simulink model "Arm_Simulation"  (R2022b)
settings: Solver=ode23t  StartTime=0.0  StopTime=10  RelTol=1e-3
undefined symbols (not defined in the file or in its folder): alpha, LF, Ts, X, Y, Z
libraries: sm_lib x16, nesl_utility x8, spsEdgeDetectorLib x6, instrumentseriallib x3, simulink_extras x3, simulink x2, svdutilitieslib x1
(part 2 of 2)

== matlab function Arm_Simulation/Path Planning/Non-Adaptive Primitive/Vertical Polynomial ==
  data: p output; t input; r_o parameter; T_swing input; beta parameter
function p = fcn(t, r_o, T_swing, beta)

T_arch = T_swing / 2;

if t <= T_arch
    % Swing Phase - Liftoff: Quintic Polynomial 1
    c0 = 0;
    c1 = 0;
    c2 = 0;
    c3 = 10 / T_arch^3;
    c4 = -15 / T_arch^4;
    c5 = 6 / T_arch^5;
    
    C = [c0; c1; c2; c3; c4; c5];
    T = [1, t, t^2, t^3, t^4, t^5];

    p = r_o*T*C;
elseif t <= T_swing
    % Swing Phase - Touchdown: Quintic Polynomial 2
    c0 = 1;
    c1 = 0;
    c2 = 0;
    c3 = -10 / T_arch^3;
    c4 = 15 / T_arch^4;
    c5 = -6 / T_arch^5;
    
    C = [c0; c1; c2; c3; c4; c5];

    t = t - T_arch;

    T = [1, t, t^2, t^3, t^4, t^5];

    p = r_o*T*C;
else
    % Stance Phase: Zero
    p = 0;
end

== matlab function Arm_Simulation/Path Planning/Non-Adaptive Primitive/Horizontal Polynomial ==
  data: p output; t input; r_o parameter; T_swing input; beta parameter
function p = fcn(t, r_o, T_swing, beta)

v = -2*r_o / beta;

offset = 2*r_o - v*T_swing;

c0 = -r_o;
c1 = v;
c2 = 0;
c3 = 10 * offset / T_swing^3;
c4 = -15 * offset / T_swing^4;
c5 = 6 * offset / T_swing^5;

C = [c0; c1; c2; c3; c4; c5];
T = [1, t, t^2, t^3, t^4, t^5];

p = T*C;

== matlab function Arm_Simulation/Path Planning/Adaptive Primitive/Vertical/Liftoff Polynomial ==
  data: p output; t input; r_o parameter; T_up input; z input
function p = fcn(t, r_o, T_up, z)

p = (r_o - z);

c0 = z;
c1 = 0;
c2 = 0;
c3 = p * 10 / T_up^3;
c4 = -p * 15 / T_up^4;
c5 = p * 6 / T_up^5;

C = [c0; c1; c2; c3; c4; c5];
T = [1, t, t^2, t^3, t^4, t^5];

p = T*C;

== matlab function Arm_Simulation/Path Planning/Adaptive Primitive/Vertical/Touchdown Polynomial ==
  data: T_up output; p output; t input; r_o parameter; delta input; beta parameter
function [T_up, p] = fcn(t, r_o, delta, beta)

T_down = (1 - beta) / 2;
T_up = T_down + delta;

% Swing Phase - Touchdown: Quintic Polynomial 2
c0 = 1;
c1 = 0;
c2 = 0;
c3 = -10 / T_down^3;
c4 = 15 / T_down^4;
c5 = -6 / T_down^5;

C = [c0; c1; c2; c3; c4; c5];

t = t - T_up;

T = [1, t, t^2, t^3, t^4, t^5];

p = r_o*T*C;

== matlab function Arm_Simulation/FK Sim/DH Row 2 ==
  data: theta input; d input; alpha input; T output; a input
function T = fcn(theta, d, alpha, a)

ct = cos(theta);
st = sin(theta);
ca = cos(alpha);
sa = sin(alpha);

T = [    ct,   -st,    0,      a;
      st*ca,  ct*ca, -sa,  -sa*d;
      st*sa,  ct*sa,  ca,   ca*d;
          0,      0,    0,      1];
end

== matlab function Arm_Simulation/FK Sim/DH Row 1 ==
  data: theta input; d input; alpha input; T output; a input
function T = fcn(theta, d, alpha, a)

ct = cos(theta);
st = sin(theta);
ca = cos(alpha);
sa = sin(alpha);

T = [    ct,   -st,    0,      a;
      st*ca,  ct*ca, -sa,  -sa*d;
      st*sa,  ct*sa,  ca,   ca*d;
          0,      0,    0,      1];
end

== matlab function Arm_Simulation/FK Sim/DH Row 3 ==
  data: theta input; d input; alpha input; T output; a input
function T = fcn(theta, d, alpha, a)

ct = cos(theta);
st = sin(theta);
ca = cos(alpha);
sa = sin(alpha);

T = [    ct,   -st,    0,      a;
      st*ca,  ct*ca, -sa,  -sa*d;
      st*sa,  ct*sa,  ca,   ca*d;
          0,      0,    0,      1];
end

== matlab function Arm_Simulation/FK Sim/DH Row 4 ==
  data: theta input; d input; alpha input; T output; a input
function T = fcn(theta, d, alpha, a)

ct = cos(theta);
st = sin(theta);
ca = cos(alpha);
sa = sin(alpha);

T = [    ct,   -st,    0,      a;
      st*ca,  ct*ca, -sa,  -sa*d;
      st*sa,  ct*sa,  ca,   ca*d;
          0,      0,    0,      1];
end

== matlab function Arm_Simulation/FK Sim1/DH Row 1 ==
  data: theta input; d input; alpha input; T output; a input
function T = fcn(theta, d, alpha, a)

ct = cos(theta);
st = sin(theta);
ca = cos(alpha);
sa = sin(alpha);

T = [    ct,   -st,    0,      a;
      st*ca,  ct*ca, -sa,  -sa*d;
      st*sa,  ct*sa,  ca,   ca*d;
          0,      0,    0,      1];
end

== matlab function Arm_Simulation/FK Sim1/DH Row 2 ==
  data: theta input; d input; alpha input; T output; a input
function T = fcn(theta, d, alpha, a)

ct = cos(theta);
st = sin(theta);
ca = cos(alpha);
sa = sin(alpha);

T = [    ct,   -st,    0,      a;
      st*ca,  ct*ca, -sa,  -sa*d;
      st*sa,  ct*sa,  ca,   ca*d;
          0,      0,    0,      1];
end

== matlab function Arm_Simulation/FK Sim1/DH Row 3 ==
  data: theta input; d input; alpha input; T output; a input
function T = fcn(theta, d, alpha, a)

ct = cos(theta);
st = sin(theta);
ca = cos(alpha);
sa = sin(alpha);

T = [    ct,   -st,    0,      a;
      st*ca,  ct*ca, -sa,  -sa*d;
      st*sa,  ct*sa,  ca,   ca*d;
          0,      0,    0,      1];
end

== matlab function Arm_Simulation/FK Sim1/DH Row 4 ==
  data: theta input; d input; alpha input; T output; a input
function T = fcn(theta, d, alpha, a)

ct = cos(theta);
st = sin(theta);
ca = cos(alpha);
sa = sin(alpha);

T = [    ct,   -st,    0,      a;
      st*ca,  ct*ca, -sa,  -sa*d;
      st*sa,  ct*sa,  ca,   ca*d;
          0,      0,    0,      1];
end

== matlab function Arm_Simulation/Path Planning/Adaptive Primitive/Horizontal/Horizontal Polynomial ==
  data: p output; t input; r_o parameter; T_swing input; beta parameter
function p = fcn(t, r_o, T_swing, beta)

v = -2*r_o / beta;

offset = 2*r_o - v*T_swing;

c0 = -r_o;
c1 = v;
c2 = 0;
c3 = 10 * offset / T_swing^3;
c4 = -15 * offset / T_swing^4;
c5 = 6 * offset / T_swing^5;

C = [c0; c1; c2; c3; c4; c5];
T = [1, t, t^2, t^3, t^4, t^5];

p = T*C;
